simulink model "Main"  (R2024b)
settings: Solver=VariableStepAuto  StartTime=0.0  StopTime=10.0  RelTol=1e-3
undefined symbols (not defined in the file): T200
libraries: shared6dof x1
settings Model: Creator=hough  LastModifiedBy=hough
settings RTWCC: GPUComputeCapability=3.5

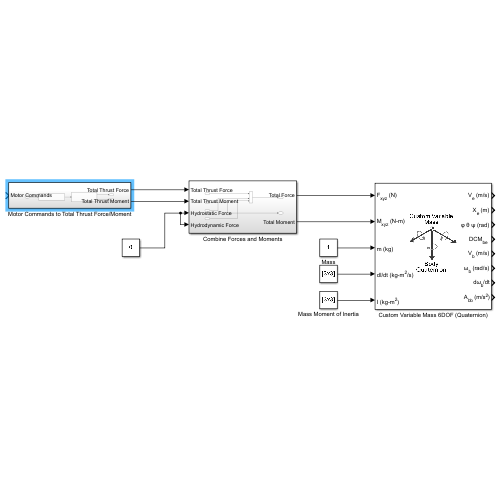
[thumbnail: Simulink's stored preview of the top-level diagram]
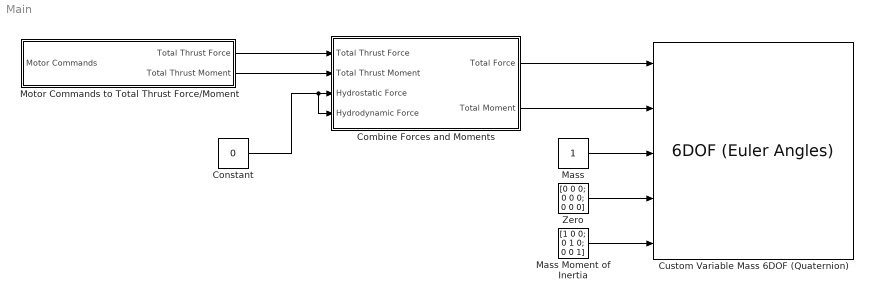
== system Main ==
  Combine Forces and Moments : Subsystem
  Constant : Constant  Value=0
  Custom Variable Mass 6DOF (Quaternion) : shared6dof/6DOF (Euler Angles)  units=Metric (MKS)  mtype=Custom Variable  rep=Quaternion  xme_0=[0 0 0]  Vm_0=[0 0 0]  eul_0=[0 0 0]  pm_0=[0 0 0]  mass_0=1.0  mass_e=0.5  mass_f=2.0  inertia=eye(3)  inertia_e=eye(3)  inertia_f=2*eye(3)  k_quat=1.0  vre_flag=off  abi_flag=off  aMode=0  xme_statename=''  Vm_statename=''  eul_statename=''  quat_statename=''  pm_statename=''  mass_statename=''
      settings: LibrarySourceBlock=aerolib6dof2/Custom Variable Mass 6DOF (Quaternion)
  Mass : Constant
  Mass Moment of Inertia : Constant  Value=[1 0 0; 0 1 0; 0 0 1]
  Motor Commands to Total Thrust Force/Moment : Subsystem
  Zero : Constant  Value=[0 0 0; 0 0 0; 0 0 0]
  wires:
  Mass/1 -> Custom Variable Mass 6DOF (Quaternion)/3
  Mass Moment of Inertia/1 -> Custom Variable Mass 6DOF (Quaternion)/5
  Zero/1 -> Custom Variable Mass 6DOF (Quaternion)/4
  Combine Forces and Moments/1(Total Force) -> Custom Variable Mass 6DOF (Quaternion)/1
  Combine Forces and Moments/2(Total Moment) -> Custom Variable Mass 6DOF (Quaternion)/2
  Motor Commands to Total Thrust Force/Moment/1(Total Thrust Force) -> Combine Forces and Moments/1(Total Thrust Force)
  Motor Commands to Total Thrust Force/Moment/2(Total Thrust Moment) -> Combine Forces and Moments/2(Total Thrust Moment)
  Constant/1 -> Combine Forces and Moments/4(Hydrodynamic Force), Combine Forces and Moments/3(Hydrostatic Force)

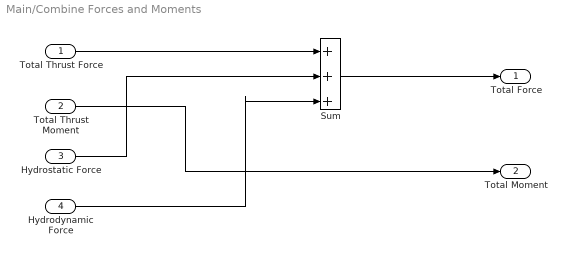
== system Main/Combine Forces and Moments ==
  Total Thrust Force : Inport
  Total Thrust Moment : Inport  Port=2
  Hydrostatic Force : Inport  Port=3
  Hydrodynamic Force : Inport  Port=4
  Sum : Sum  Inputs=+|++
  Total Force : Outport
  Total Moment : Outport  Port=2
  wires:
  Sum/1 -> Total Force/1
  Total Thrust Force/1 -> Sum/1
  Hydrostatic Force/1 -> Sum/2
  Hydrodynamic Force/1 -> Sum/3
  Total Thrust Moment/1 -> Total Moment/1

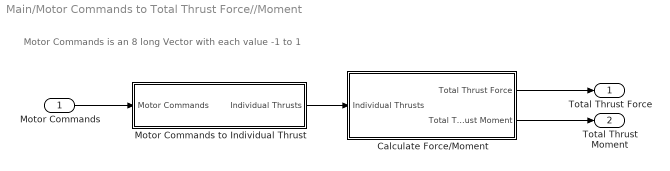
== system Main/Motor Commands to Total Thrust Force//Moment ==
  note: Motor Commands is an 8 long Vector with each value -1 to 1
  Motor Commands : Inport
  Calculate Force/Moment : Subsystem
  Motor Commands to Individual Thrust : Subsystem
  Total Thrust Force : Outport
  Total Thrust Moment : Outport  Port=2
  wires:
  Motor Commands/1 -> Motor Commands to Individual Thrust/1(Motor Commands)
  Calculate Force/Moment/1(Total Thrust Force) -> Total Thrust Force/1
  Calculate Force/Moment/2(Total Thrust Moment) -> Total Thrust Moment/1
  Motor Commands to Individual Thrust/1(Individual Thrusts) -> Calculate Force/Moment/1(Individual Thrusts)

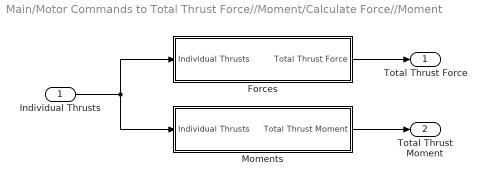
== system Main/Motor Commands to Total Thrust Force//Moment/Calculate Force//Moment ==
  Individual Thrusts : Inport
  Forces : Subsystem
  Moments : Subsystem
  Total Thrust Force : Outport
  Total Thrust Moment : Outport  Port=2
  wires:
  Individual Thrusts/1 -> Forces/1(Individual Thrusts), Moments/1(Individual Thrusts)
  Forces/1(Total Thrust Force) -> Total Thrust Force/1
  Moments/1(Total Thrust Moment) -> Total Thrust Moment/1

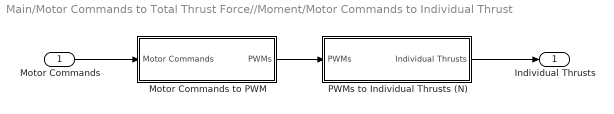
== system Main/Motor Commands to Total Thrust Force//Moment/Motor Commands to Individual Thrust ==
  Motor Commands : Inport
  Motor Commands to PWM : Subsystem
  PWMs to Individual Thrusts (N) : Subsystem
  Individual Thrusts : Outport
  wires:
  Motor Commands/1 -> Motor Commands to PWM/1(Motor Commands)
  Motor Commands to PWM/1(PWMs) -> PWMs to Individual Thrusts (N)/1(PWMs)
  PWMs to Individual Thrusts (N)/1(Individual Thrusts) -> Individual Thrusts/1

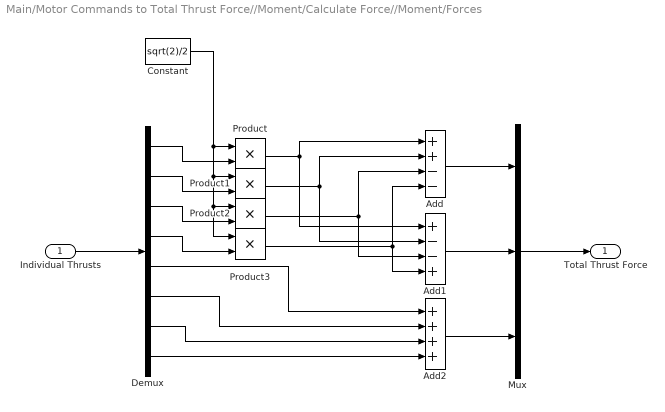
== system Main/Motor Commands to Total Thrust Force//Moment/Calculate Force//Moment/Forces ==
  Individual Thrusts : Inport
  Add : Sum  Inputs=++--
  Add1 : Sum  Inputs=+--+
  Add2 : Sum  Inputs=++++
  Constant : Constant  Value=sqrt(2)/2
  Demux : Demux  Outputs=8
  Mux : Mux  Inputs=3
  Product{,1..3} (4 alike) : Product
  Total Thrust Force : Outport
  wires:
  Individual Thrusts/1 -> Demux/1
  Add/1 -> Mux/1
  Add1/1 -> Mux/2
  Constant/1 -> Product3/1, Product2/1, Product1/1, Product/1
  Demux/1 -> Product/2
  Demux/2 -> Product1/2
  Demux/3 -> Product2/2
  Demux/4 -> Product3/2
  Demux/5 -> Add2/1
  Demux/6 -> Add2/2
  Demux/7 -> Add2/3
  Demux/8 -> Add2/4
  Product/1 -> Add/1, Add1/1
  Product1/1 -> Add/2, Add1/2
  Product2/1 -> Add/3, Add1/3
  Product3/1 -> Add/4, Add1/4
  Add2/1 -> Mux/3
  Mux/1 -> Total Thrust Force/1

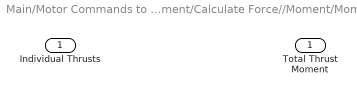
== system Main/Motor Commands to Total Thrust Force//Moment/Calculate Force//Moment/Moments ==
  Individual Thrusts : Inport
  Total Thrust Moment : Outport

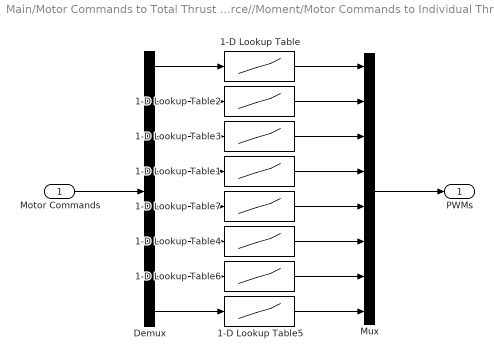
== system Main/Motor Commands to Total Thrust Force//Moment/Motor Commands to Individual Thrust/Motor Commands to PWM ==
  Motor Commands : Inport
  1-D Lookup Table{,1..7} (8 alike) : Lookup_n-D  NumberOfTableDimensions=1  BreakpointsForDimension1=[-1:0.01:1]  Table=1500 + 400*[-1:0.01:1]  InternalRulePriority=Speed  RndMeth=Simplest
  Demux : Demux  Outputs=8
  Mux : Mux  Inputs=8
  PWMs : Outport
  wires:
  Motor Commands/1 -> Demux/1
  Mux/1 -> PWMs/1
  Demux/1 -> 1-D Lookup Table/1
  Demux/2 -> 1-D Lookup Table2/1
  Demux/3 -> 1-D Lookup Table3/1
  Demux/4 -> 1-D Lookup Table1/1
  Demux/5 -> 1-D Lookup Table7/1
  Demux/6 -> 1-D Lookup Table4/1
  Demux/7 -> 1-D Lookup Table6/1
  Demux/8 -> 1-D Lookup Table5/1
  1-D Lookup Table/1 -> Mux/1
  1-D Lookup Table2/1 -> Mux/2
  1-D Lookup Table3/1 -> Mux/3
  1-D Lookup Table1/1 -> Mux/4
  1-D Lookup Table4/1 -> Mux/6
  1-D Lookup Table7/1 -> Mux/5
  1-D Lookup Table6/1 -> Mux/7
  1-D Lookup Table5/1 -> Mux/8

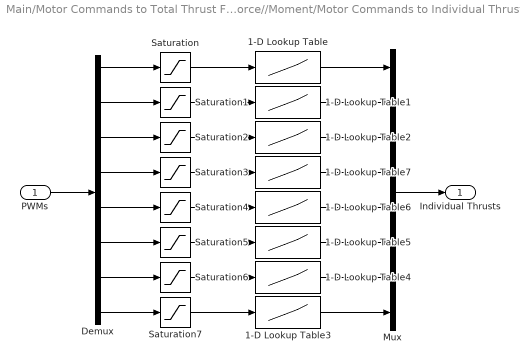
== system Main/Motor Commands to Total Thrust Force//Moment/Motor Commands to Individual Thrust/PWMs to Individual Thrusts (N) ==
  PWMs : Inport
  1-D Lookup Table{,1..7} (8 alike) : Lookup_n-D  NumberOfTableDimensions=1  BreakpointsForDimension1=1500 + 400*[-1:0.01:1]  Table=T200{:,2}'  InternalRulePriority=Speed  RndMeth=Simplest
  Demux : Demux  Outputs=8
  Mux : Mux  Inputs=8
  Saturation{,1..7} (8 alike) : Saturate  UpperLimit=1900  LowerLimit=1100
  Individual Thrusts : Outport
  wires:
  Mux/1 -> Individual Thrusts/1
  PWMs/1 -> Demux/1
  Demux/1 -> Saturation/1
  Demux/2 -> Saturation1/1
  Demux/3 -> Saturation2/1
  Demux/4 -> Saturation3/1
  Demux/5 -> Saturation4/1
  Demux/6 -> Saturation5/1
  Demux/7 -> Saturation6/1
  Demux/8 -> Saturation7/1
  Saturation/1 -> 1-D Lookup Table/1
  Saturation1/1 -> 1-D Lookup Table1/1
  Saturation2/1 -> 1-D Lookup Table2/1
  Saturation3/1 -> 1-D Lookup Table7/1
  Saturation4/1 -> 1-D Lookup Table6/1
  Saturation5/1 -> 1-D Lookup Table5/1
  Saturation6/1 -> 1-D Lookup Table4/1
  Saturation7/1 -> 1-D Lookup Table3/1
  1-D Lookup Table/1 -> Mux/1
  1-D Lookup Table1/1 -> Mux/2
  1-D Lookup Table2/1 -> Mux/3
  1-D Lookup Table7/1 -> Mux/4
  1-D Lookup Table6/1 -> Mux/5
  1-D Lookup Table5/1 -> Mux/6
  1-D Lookup Table4/1 -> Mux/7
  1-D Lookup Table3/1 -> Mux/8
